simulink library "Copy_of_PTOSim_Lib"  (R2014b)
settings: Solver=ode45  StartTime=0.0  StopTime=10.0  RelTol=1e-3
undefined symbols (not defined in the file or in its folder): pAeq, pAupper_limit, pBeq, pBupper_limit, ptosim, tot
undefined symbols (not defined in the file): valve
settings Model: RequirementInfo="{}  %GIDa_42666abb_d6d9_408c_ae24_f6520282b61c"  Creator=sor  LastModifiedBy=rso

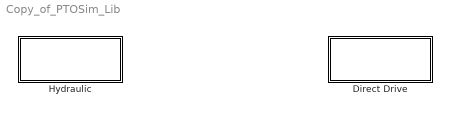
== system Copy_of_PTOSim_Lib ==
  Direct Drive : Subsystem  RequirementInfo="{}  %GIDa_5439fdb4_7c29_433c_8677_23bf92e18f11"
  Hydraulic : Subsystem  RequirementInfo={} %GIDa_f12a42eb_b9cb_4818_b573_b7dee4183a3b

== system Copy_of_PTOSim_Lib/Direct Drive ==
  Electric Machine : Subsystem  RequirementInfo="{}  %GIDa_9a577bd3_d1cd_44c9_a605_4eaf21e33064"  mask{ptosim=ptosim.machine}
      mask prompts: ptosim "Machine Name:"
      mask init:
      | if exist ('ptosim','var')
      |     if ischar(ptosim.Rs)==1 ...
      |        || ischar(ptosim.Bfric)==1 ...
      |        || ischar(ptosim.tau_p)==1 ...
      |        || ischar(ptosim.lambda_fd)==1 ...
      |        || ischar(ptosim.Ls)==1 ...
      |        || ischar(ptosim.theta_d_0)==1 ...
      |        || ischar(ptosim.lambda_sq_0)==1 ...
      |        || ischar(ptosim.lambda_sd_0)==1
      |           error('One of the machine variables is undefined. For example, ptosim.machine.variableName')
      |     end       
      | end
  Load : Subsystem  mask(PTO-Sim Element){ptosim=ptosim.ddload}
      mask prompts: ptosim "Load Name:"
      mask init:
      | if exist ('ptosim','var')
      |     if ischar(ptosim.Rload)==1
      |         error('ptosim.ddload.Rload is undefined')
      |     end
      | end

== system Copy_of_PTOSim_Lib/Hydraulic ==
  Accumulator : Subsystem  mask(PTO-Sim Element){ptosim=ptosim}
      mask prompts: ptosim "Accumulator Name:"
      mask init:
      | if exist('ptosim','var')
      |     if ischar(ptosim.VI0)==1 ...
      |             || ischar(ptosim.pIrated)==1 ...
      |             || ischar(ptosim.pIupper_limit)==1 ...
      |             || ischar(ptosim.pIlower_limit)==1 ...
      |             || ischar(ptosim.pIprecharge)==1 ...
      |             || ischar(ptosim.VImax)==1 ...
      |             || ischar(ptosim.VImin)==1 ...
      |             || ischar(ptosim.VIeq)==1 ...
      |             || ischar(ptosim.pIeq)==1 ...
      |             error('One of the accumulator variable is undefined. For example, ptosim.accum.variableName')
      |     end
      | end
  "Hydraulic Motor " : Subsystem  mask{ptosim=ptosim.motor}
      mask prompts: ptosim "Motor Name:"
      mask init:
      | if exist ('ptosim','var')
      |     if ischar(ptosim.angVelInit)==1 ...
      |        || ischar(ptosim.alpha)==1 ...
      |        || ischar(ptosim.D)==1 ...
      |        || ischar(ptosim.J)==1 ...
      |        || ischar(ptosim.bg)==1 ...
      |        || ischar(ptosim.bf)==1
      |           error('One of the motor variables is undefined. For example, ptosim.motor.variableName')
      |     end       
      | end
  Lookup Table Generator : Subsystem  RequirementInfo="{}  %GIDa_30368e1c_dc2a_4605_bb50_ff3a423f2df5"  mask{ptosim=ptosim.gen}
      mask prompts: ptosim "Generator Name"
      mask init:
      | if exist ('ptosim','var')
      |    if ischar(ptosim.TgenBase)==1 ...
      |       || ischar(ptosim.omegaBase)==1 ...
      |       || ischar(ptosim.driveEff)==1 
      |          error('One of the generator variables is undefined. For example, ptosim.gen.variableName')
      |    end
      | end
  Piston : Subsystem  Variant=on  mask(PTO-Element){piston=ptosim.piston}
      mask prompts: piston "Piston Name:"
  Valve : Subsystem  Variant=on  mask{valve=valve}
      mask prompts: valve "Valve Name"

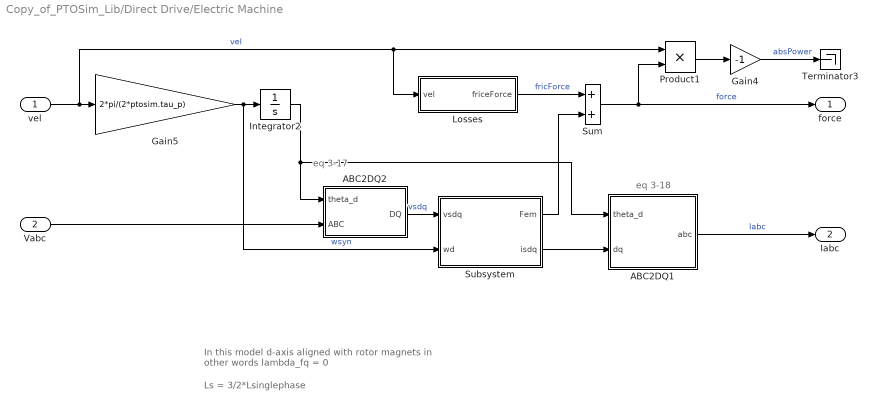
== system Copy_of_PTOSim_Lib/Direct Drive/Electric Machine ==
  note: In this model d-axis aligned with rotor magnets
      | in other words lambda_fq = 0
  note: Ls = 3/2*Lsinglephase
  note: eq 3-17
  note: eq 3-18
  vel : Inport
  Vabc : Inport  Port=2
  ABC2DQ1 : Subsystem
  ABC2DQ2 : Subsystem
  Gain4 : Gain  Gain=-1
  Gain5 : Gain  Gain=2*pi/(2*ptosim.tau_p)
  Integrator2 : Integrator  InitialCondition=ptosim.theta_d_0
  Losses : Subsystem
  Product1 : Product
  Subsystem : Subsystem
  Sum : Sum
  Terminator3 : Terminator
  force : Outport
  Iabc : Outport  Port=2
  wires:
  ABC2DQ2/1(DQ) -> Subsystem/1(vsdq)  "vsdq"
  ABC2DQ1/1(abc) -> Iabc/1  "Iabc"
  vel/1 -> Gain5/1, Losses/1(vel), Product1/1  "vel"
  Gain5/1 -> Subsystem/2(wd), Integrator2/1  "wsyn"
  Integrator2/1 -> ABC2DQ2/1(theta_d), ABC2DQ1/1(theta_d)
  Product1/1 -> Gain4/1
  Gain4/1 -> Terminator3/1  "absPower"
  Subsystem/1(Fem) -> Sum/2
  Vabc/1 -> ABC2DQ2/2(ABC)
  Subsystem/2(isdq) -> ABC2DQ1/2(dq)
  Losses/1(friceForce) -> Sum/1  "fricForce"
  Sum/1 -> Product1/2, force/1  "force"

== system Copy_of_PTOSim_Lib/Direct Drive/Load ==
  Iabc : Inport
  Gain : Gain  Gain=-1
  Gain1 : Gain  Gain=ptosim.Rload
  Product : Product
  Sum of Elements : Sum  Inputs=+
  Vabc : Outport
  elecPower : Outport  Port=2
  wires:
  Gain/1 -> elecPower/1  "elecPower"
  Gain1/1 -> Product/1, Vabc/1  "Vabc"
  Product/1 -> Sum of Elements/1
  Iabc/1 -> Gain1/1, Product/2
  Sum of Elements/1 -> Gain/1

== system Copy_of_PTOSim_Lib/Hydraulic/Accumulator ==
  volFlowM : Inport
  volFlowAccum : Inport  Port=2
  Constant : Constant
  Constant3 : Constant  Value=ptosim.pIprecharge
  Constant4 : Constant  Value=ptosim.VI0
  Divide : Product  Inputs=*/
  Divide1 : Product  Inputs=*/
  Exponent : Constant  Value=1.4
  Integrator4 : Integrator  InitialCondition=ptosim.VIeq
  Math Function : Math  Operator=pow  SaturateOnIntegerOverflow=on
  Sum : Sum  Inputs=-+
  Sum2 : Sum
  pressure : Outport
  wires:
  Sum2/1 -> Integrator4/1
  Integrator4/1 -> Divide/1
  Constant4/1 -> Divide/2
  Constant/1 -> Sum/2
  Divide/1 -> Sum/1
  Exponent/1 -> Math Function/2
  Sum/1 -> Math Function/1
  Math Function/1 -> Divide1/2
  Constant3/1 -> Divide1/1  "pI0"
  Divide1/1 -> pressure/1
  volFlowAccum/1 -> Sum2/2
  volFlowM/1 -> Sum2/1

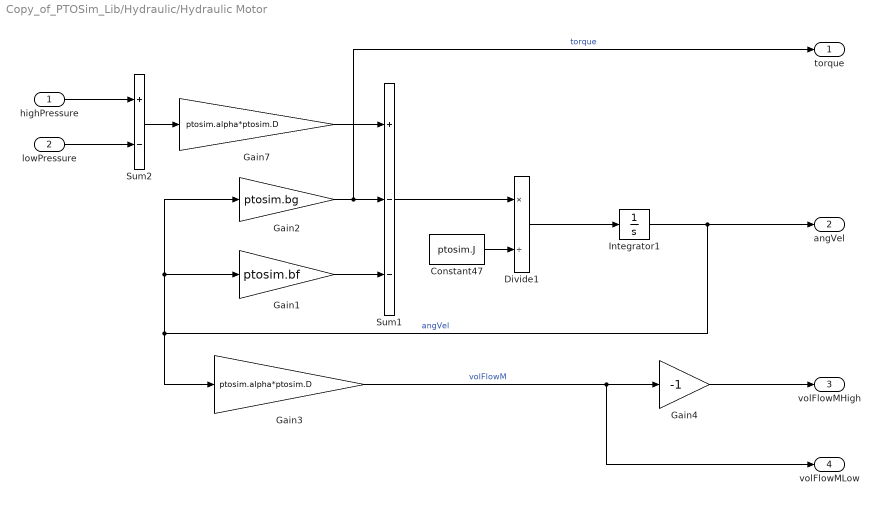
== system Copy_of_PTOSim_Lib/Hydraulic/Hydraulic Motor  ==
  highPressure : Inport
  lowPressure : Inport  Port=2
  Constant47 : Constant  Value=ptosim.J
  Divide1 : Product  Inputs=*/
  Gain1 : Gain  Gain=ptosim.bf
  Gain2 : Gain  Gain=ptosim.bg
  Gain3 : Gain  Gain=ptosim.alpha*ptosim.D
  Gain4 : Gain  Gain=-1
  Gain7 : Gain  Gain=ptosim.alpha*ptosim.D
  Integrator1 : Integrator  InitialCondition=ptosim.angVelInit
  Sum1 : Sum  Inputs=+--
  Sum2 : Sum  Inputs=+-
  torque : Outport
  angVel : Outport  Port=2
  volFlowMHigh : Outport  Port=3
  volFlowMLow : Outport  Port=4
  wires:
  Gain7/1 -> Sum1/1
  Gain2/1 -> torque/1, Sum1/2  "torque"
  Gain1/1 -> Sum1/3
  Sum1/1 -> Divide1/1
  Constant47/1 -> Divide1/2
  Divide1/1 -> Integrator1/1
  Integrator1/1 -> angVel/1, Gain3/1, Gain2/1, Gain1/1  "angVel"
  Gain3/1 -> volFlowMLow/1, Gain4/1  "volFlowM"
  highPressure/1 -> Sum2/1
  lowPressure/1 -> Sum2/2
  Sum2/1 -> Gain7/1
  Gain4/1 -> volFlowMHigh/1

== system Copy_of_PTOSim_Lib/Hydraulic/Lookup Table Generator ==
  torque : Inport
  angVel : Inport  Port=2
  Base Motor Torque : Gain  Gain=-1/ptosim.TgenBase
  Base Motor Torque1 : Gain  Gain=1/ptosim.omegaBase
  Base Motor Torque2 : Gain  Gain=ptosim.driveEff
  Base Motor Torque3 : Gain  Gain=1/100
  PM p.u. Efficiency Lookup Table : Lookup_n-D  BreakpointsForDimension1=tot.Tpu(:,1)  BreakpointsForDimension2=tot.omegapu(1,:)  Table=tot.eff  InterpMethod=Flat  InputSameDT=on
  Product : Product  RndMeth=Zero
  Product1 : Product  RndMeth=Zero
  elecPower : Outport
  wires:
  Base Motor Torque2/1 -> elecPower/1  "elecPower"
  Product1/1 -> Base Motor Torque2/1
  Product/1 -> Product1/1  "genPower"
  Base Motor Torque3/1 -> Product1/2  "genEff"
  PM p.u. Efficiency Lookup Table/1 -> Base Motor Torque3/1
  angVel/1 -> Product/2, Base Motor Torque1/1
  Base Motor Torque1/1 -> PM p.u. Efficiency Lookup Table/2  "omegaPU"
  torque/1 -> Product/1, Base Motor Torque/1
  Base Motor Torque/1 -> PM p.u. Efficiency Lookup Table/1  "torquePU"

== system Copy_of_PTOSim_Lib/Hydraulic/Piston ==
  note: 1) Add Subsystem or Model blocks as valid variant choices.
      | 2) You cannot connect blocks at this level. At simulation, connectivity is automatically
      | determined, based on the active variant and port name matching.
  response : Inport
  volFlowC : Inport  Port=2
  pressureNC : Inport  Port=3
  PistonC : Subsystem  VariantControl=compressFluid  mask{ptosim=ptosim.piston}
      mask prompts: ptosim "Piston Name:"
      mask init:
      | if exist ('ptosim','var')
      |     if ischar(ptosim.Ap)==1 ...
      |       || ischar(ptosim.Vo)==1 ...
      |       || ischar(ptosim.Beta_e)==1 ...
      |       || ischar(ptosim.pAi)==1 ...
      |       || ischar(ptosim.pBi)==1 
      |          error('One of the piston variable is undefined. For example, ptosim.piston.variableName')    
      |     end
      | end
  PistonNC : Subsystem  VariantControl=noncompressFluid  mask(PTO-Sim Element){ptosim=ptosim.piston}
      mask prompts: ptosim "Piston Name:"
      mask init:
      | if exist ('ptosim','var')
      |     if ischar(ptosim.topA)==1 ...
      |       || ischar(ptosim.botA)==1
      |          error('One of the piston variables is undefined. For example, ptosim.piston.variableName')
      |     end
      | end
  force : Outport
  pressureC : Outport  Port=2
  volFlowNC : Outport  Port=3

== system Copy_of_PTOSim_Lib/Hydraulic/Valve ==
  note: 1) Add Subsystem or Model blocks as valid variant choices.
      | 2) You cannot connect blocks at this level. At simulation, connectivity is automatically
      | determined, based on the active variant and port name matching.
  pressureC : Inport
  volFlowNC : Inport  Port=2
  ValveC : Subsystem  VariantControl=compressFluid  mask{ptosim=ptosim.valve}
      mask prompts: ptosim "Valve Name:"
      mask init:
      | if exist ('ptosim','var')
      |     if ischar(ptosim.Cd)==1 ...
      |        || ischar(ptosim.Amax)==1 ...
      |        || ischar(ptosim.Amin)==1 ...
      |        || ischar(ptosim.pMax)==1 ...
      |        || ischar(ptosim.pMin)==1 ...
      |        || ischar(ptosim.rho)==1 ...
      |        || ischar(ptosim.k1)==1 ...
      |        || ischar(ptosim.k2)==1 
      |           error('One of valve variables is undefined. For exmaple, ptosim.valve.variableName')
      |     end
      | end
  ValveNC : Subsystem  VariantControl=noncompressFluid  mask(PTO-Sim Element){ptosim=0}
      mask prompts: ptosim "Valve Name:"
  volFlow : Outport

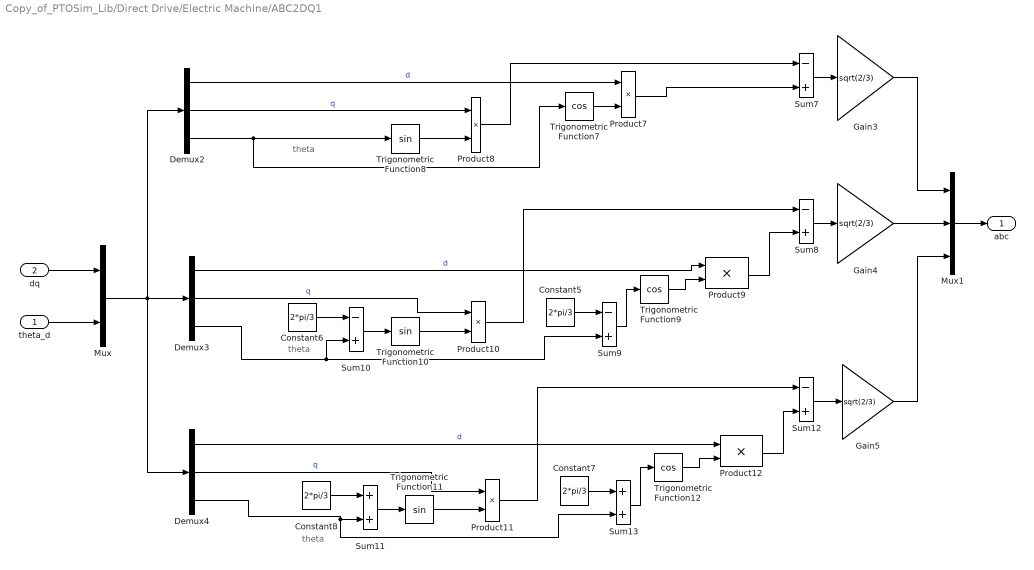
== system Copy_of_PTOSim_Lib/Direct Drive/Electric Machine/ABC2DQ1 ==
  note: theta
  note: theta
  note: theta
  theta_d : Inport
  dq : Inport  Port=2
  Constant{5..8} (4 alike) : Constant  Value=2*pi/3
  Demux2 : Demux  Outputs=3
  Demux3 : Demux  Outputs=3
  Demux4 : Demux  Outputs=3
  Gain3 : Gain  Gain=sqrt(2/3)  SaturateOnIntegerOverflow=on  OutDataTypeStr=Inherit: Same as input  ParamDataTypeStr=Inherit: Same as input
  Gain4 : Gain  Gain=sqrt(2/3)  SaturateOnIntegerOverflow=on  OutDataTypeStr=Inherit: Same as input  ParamDataTypeStr=Inherit: Same as input
  Gain5 : Gain  Gain=sqrt(2/3)  SaturateOnIntegerOverflow=on  OutDataTypeStr=Inherit: Same as input  ParamDataTypeStr=Inherit: Same as input
  Mux : Mux  Inputs=2
  Mux1 : Mux  Inputs=3
  Product{7..12} (6 alike) : Product  SaturateOnIntegerOverflow=on  InputSameDT=on  OutDataTypeStr=Inherit: Same as first input
  Sum{7..10,12} (5 alike) : Sum  Inputs=-+  SaturateOnIntegerOverflow=on  InputSameDT=on  OutDataTypeStr=Inherit: Same as first input
  Sum11 : Sum  SaturateOnIntegerOverflow=on  InputSameDT=on  OutDataTypeStr=Inherit: Same as first input
  Sum13 : Sum  SaturateOnIntegerOverflow=on  InputSameDT=on  OutDataTypeStr=Inherit: Same as first input
  Trigonometric Function10 : Trigonometry
  Trigonometric Function11 : Trigonometry
  Trigonometric Function12 : Trigonometry  Operator=cos
  Trigonometric Function7 : Trigonometry  Operator=cos
  Trigonometric Function8 : Trigonometry
  Trigonometric Function9 : Trigonometry  Operator=cos
  abc : Outport
  wires:
  Mux1/1 -> abc/1
  dq/1 -> Mux/1
  theta_d/1 -> Mux/2
  Mux/1 -> Demux4/1, Demux2/1, Demux3/1
  Trigonometric Function7/1 -> Product7/2
  Demux2/1 -> Product7/1  "d"
  Product7/1 -> Sum7/2
  Product8/1 -> Sum7/1
  Demux2/3 -> Trigonometric Function8/1, Trigonometric Function7/1
  Demux2/2 -> Product8/1  "q"
  Trigonometric Function9/1 -> Product9/2
  Demux3/1 -> Product9/1  "d"
  Product9/1 -> Sum8/2
  Product10/1 -> Sum8/1
  Demux3/3 -> Sum10/2, Sum9/2
  Trigonometric Function10/1 -> Product10/2
  Demux3/2 -> Product10/1  "q"
  Sum9/1 -> Trigonometric Function9/1
  Constant5/1 -> Sum9/1
  Sum10/1 -> Trigonometric Function10/1
  Constant6/1 -> Sum10/1
  Trigonometric Function12/1 -> Product12/2
  Demux4/1 -> Product12/1  "d"
  Product12/1 -> Sum12/2
  Product11/1 -> Sum12/1
  Demux4/3 -> Sum13/2, Sum11/2
  Trigonometric Function11/1 -> Product11/2
  Demux4/2 -> Product11/1  "q"
  Sum13/1 -> Trigonometric Function12/1
  Constant7/1 -> Sum13/1
  Sum11/1 -> Trigonometric Function11/1
  Constant8/1 -> Sum11/1
  Sum7/1 -> Gain3/1
  Sum8/1 -> Gain4/1
  Sum12/1 -> Gain5/1
  Gain3/1 -> Mux1/1
  Gain4/1 -> Mux1/2
  Gain5/1 -> Mux1/3
  Trigonometric Function8/1 -> Product8/2

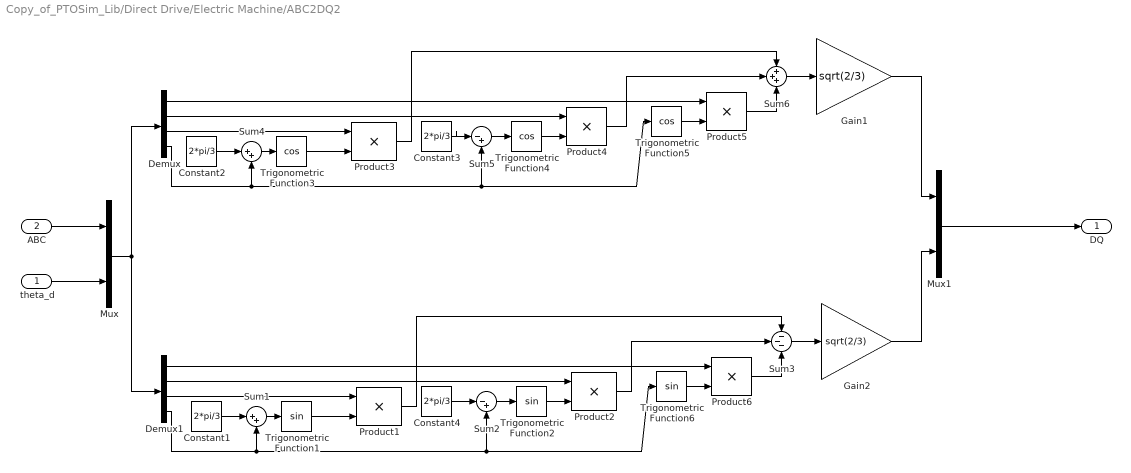
== system Copy_of_PTOSim_Lib/Direct Drive/Electric Machine/ABC2DQ2 ==
  theta_d : Inport
  ABC : Inport  Port=2
  Constant{1..4} (4 alike) : Constant  Value=2*pi/3
  Demux : Demux
  Demux1 : Demux
  Gain1 : Gain  Gain=sqrt(2/3)  SaturateOnIntegerOverflow=on  OutDataTypeStr=Inherit: Same as input  ParamDataTypeStr=Inherit: Same as input
  Gain2 : Gain  Gain=sqrt(2/3)  SaturateOnIntegerOverflow=on  OutDataTypeStr=Inherit: Same as input  ParamDataTypeStr=Inherit: Same as input
  Mux : Mux  Inputs=2
  Mux1 : Mux  Inputs=2
  Product{1..6} (6 alike) : Product  SaturateOnIntegerOverflow=on  InputSameDT=on  OutDataTypeStr=Inherit: Same as first input
  Sum1 : Sum  Inputs=|++  SaturateOnIntegerOverflow=on  InputSameDT=on  OutDataTypeStr=Inherit: Same as first input
  Sum2 : Sum  Inputs=|-+  SaturateOnIntegerOverflow=on  InputSameDT=on  OutDataTypeStr=Inherit: Same as first input
  Sum3 : Sum  Inputs=---  SaturateOnIntegerOverflow=on  InputSameDT=on  OutDataTypeStr=Inherit: Same as first input
  Sum4 : Sum  Inputs=|++  SaturateOnIntegerOverflow=on  InputSameDT=on  OutDataTypeStr=Inherit: Same as first input
  Sum5 : Sum  Inputs=|-+  SaturateOnIntegerOverflow=on  InputSameDT=on  OutDataTypeStr=Inherit: Same as first input
  Sum6 : Sum  Inputs=+++  SaturateOnIntegerOverflow=on  InputSameDT=on  OutDataTypeStr=Inherit: Same as first input
  Trigonometric Function1 : Trigonometry
  Trigonometric Function2 : Trigonometry
  Trigonometric Function3 : Trigonometry  Operator=cos
  Trigonometric Function4 : Trigonometry  Operator=cos
  Trigonometric Function5 : Trigonometry  Operator=cos
  Trigonometric Function6 : Trigonometry
  DQ : Outport
  wires:
  Mux1/1 -> DQ/1
  Product5/1 -> Sum6/3
  Constant2/1 -> Sum4/1
  Sum5/1 -> Trigonometric Function4/1
  Trigonometric Function4/1 -> Product4/2
  Trigonometric Function5/1 -> Product5/2
  Constant3/1 -> Sum5/1
  Sum6/1 -> Gain1/1
  Product3/1 -> Sum6/1
  Product4/1 -> Sum6/2
  Trigonometric Function3/1 -> Product3/2
  Gain1/1 -> Mux1/1
  ABC/1 -> Mux/1
  theta_d/1 -> Mux/2
  Demux/1 -> Product5/1
  Demux/2 -> Product4/1
  Demux/3 -> Product3/1
  Demux/4 -> Sum5/2, Trigonometric Function5/1, Sum4/2
  Mux/1 -> Demux/1, Demux1/1
  Sum4/1 -> Trigonometric Function3/1
  Product6/1 -> Sum3/3
  Constant1/1 -> Sum1/1
  Sum2/1 -> Trigonometric Function2/1
  Trigonometric Function2/1 -> Product2/2
  Trigonometric Function6/1 -> Product6/2
  Constant4/1 -> Sum2/1
  Sum3/1 -> Gain2/1
  Product1/1 -> Sum3/1
  Product2/1 -> Sum3/2
  Trigonometric Function1/1 -> Product1/2
  Gain2/1 -> Mux1/2
  Demux1/1 -> Product6/1
  Demux1/2 -> Product2/1
  Demux1/3 -> Product1/1
  Demux1/4 -> Sum1/2, Trigonometric Function6/1, Sum2/2
  Sum1/1 -> Trigonometric Function1/1

== system Copy_of_PTOSim_Lib/Direct Drive/Electric Machine/Losses ==
  vel : Inport
  Gain : Gain  Gain=ptosim.Bfric
  friceForce : Outport
  wires:
  vel/1 -> Gain/1
  Gain/1 -> friceForce/1

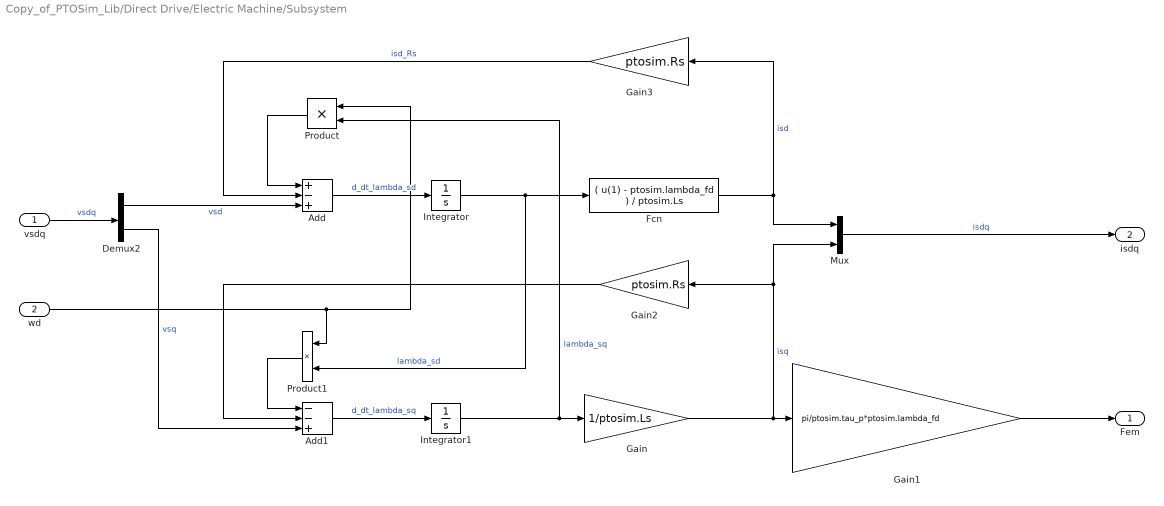
== system Copy_of_PTOSim_Lib/Direct Drive/Electric Machine/Subsystem ==
  vsdq : Inport
  wd : Inport  Port=2
  Add : Sum  Inputs=+-+
  Add1 : Sum  Inputs=--+
  Demux2 : Demux  Outputs=2
  Fcn : Fcn  Expr=( u(1) - ptosim.lambda_fd ) / ptosim.Ls
  Gain : Gain  Gain=1/ptosim.Ls
  Gain1 : Gain  Gain=pi/ptosim.tau_p*ptosim.lambda_fd
  Gain2 : Gain  Gain=ptosim.Rs
  Gain3 : Gain  Gain=ptosim.Rs
  Integrator : Integrator  InitialCondition=ptosim.lambda_sd_0
  Integrator1 : Integrator  InitialCondition=ptosim.lambda_sq_0
  Mux : Mux  Inputs=2
  Product : Product  RndMeth=Zero
  Product1 : Product  RndMeth=Zero
  Fem : Outport
  isdq : Outport  Port=2
  wires:
  Add/1 -> Integrator/1  "d_dt_lambda_sd"
  Integrator/1 -> Product1/2, Fcn/1  "lambda_sd"
  Fcn/1 -> Gain3/1, Mux/1  "isd"
  Product/1 -> Add/1
  Add1/1 -> Integrator1/1  "d_dt_lambda_sq"
  Integrator1/1 -> Gain/1, Product/2  "lambda_sq"
  wd/1 -> Product1/1, Product/1
  Gain/1 -> Gain2/1, Mux/2, Gain1/1  "isq"
  Product1/1 -> Add1/1
  Demux2/1 -> Add/3  "vsd"
  Demux2/2 -> Add1/3  "vsq"
  vsdq/1 -> Demux2/1  "vsdq"
  Gain3/1 -> Add/2  "isd_Rs"
  Gain2/1 -> Add1/2
  Mux/1 -> isdq/1  "isdq"
  Gain1/1 -> Fem/1

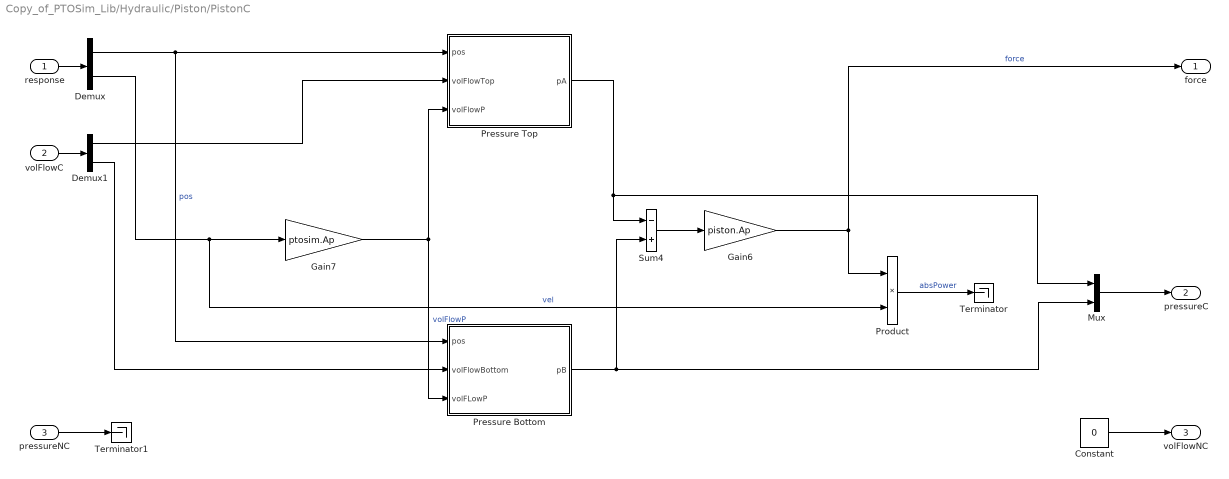
== system Copy_of_PTOSim_Lib/Hydraulic/Piston/PistonC ==
  response : Inport
  volFlowC : Inport  Port=2
  pressureNC : Inport  Port=3
  Constant : Constant  Value=0
  Demux : Demux  Outputs=2
  Demux1 : Demux  Outputs=2
  Gain6 : Gain  Gain=piston.Ap
  Gain7 : Gain  Gain=ptosim.Ap
  Mux : Mux  Inputs=2
  Pressure Bottom : Subsystem
  Pressure Top : Subsystem
  Product : Product
  Sum4 : Sum  Inputs=-+
  Terminator : Terminator
  Terminator1 : Terminator
  force : Outport
  pressureC : Outport  Port=2
  volFlowNC : Outport  Port=3
  wires:
  Pressure Top/1(pA) -> Mux/1, Sum4/1
  Pressure Bottom/1(pB) -> Mux/2, Sum4/2
  Gain7/1 -> Pressure Bottom/3(volFLowP), Pressure Top/3(volFlowP)  "volFlowP"
  Product/1 -> Terminator/1  "absPower"
  Demux/1 -> Pressure Bottom/1(pos), Pressure Top/1(pos)  "pos"
  Demux/2 -> Product/2, Gain7/1  "vel"
  Sum4/1 -> Gain6/1
  Gain6/1 -> force/1, Product/1  "force"
  Demux1/1 -> Pressure Top/2(volFlowTop)
  Demux1/2 -> Pressure Bottom/2(volFlowBottom)
  response/1 -> Demux/1
  volFlowC/1 -> Demux1/1
  Mux/1 -> pressureC/1
  Constant/1 -> volFlowNC/1
  pressureNC/1 -> Terminator1/1

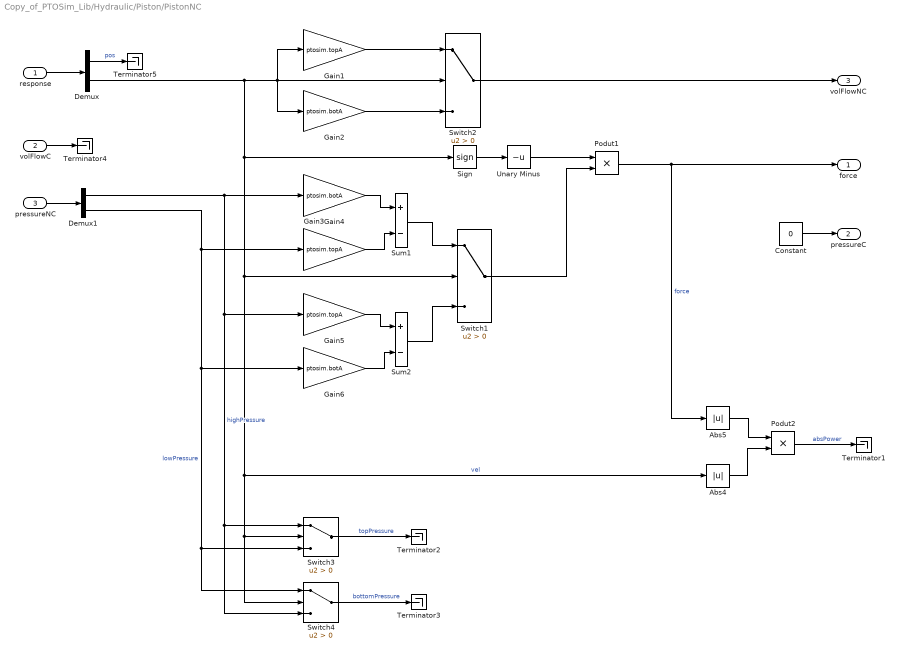
== system Copy_of_PTOSim_Lib/Hydraulic/Piston/PistonNC ==
  response : Inport
  volFlowC : Inport  Port=2
  pressureNC : Inport  Port=3
  Abs4 : Abs
  Abs5 : Abs
  Constant : Constant  Value=0
  Demux : Demux  Outputs=2
  Demux1 : Demux  Outputs=2
  Gain1 : Gain  Gain=ptosim.topA
  Gain2 : Gain  Gain=ptosim.botA
  Gain3 : Gain  Gain=ptosim.topA
  Gain4 : Gain  Gain=ptosim.botA
  Gain5 : Gain  Gain=ptosim.topA
  Gain6 : Gain  Gain=ptosim.botA
  Podut1 : Product  RndMeth=Zero
  Podut2 : Product  RndMeth=Zero
  Sign : Signum
  Sum1 : Sum  Inputs=+-
  Sum2 : Sum  Inputs=+-
  Switch{1..4} (4 alike) : Switch  Criteria=u2 > Threshold
  Terminator{1..5} (5 alike) : Terminator
  Unary Minus : UnaryMinus
  force : Outport
  pressureC : Outport  Port=2
  volFlowNC : Outport  Port=3
  wires:
  Demux/2 -> Switch1/2, Switch4/2, Switch3/2, Abs4/1, Sign/1, Gain2/1, Switch2/2, Gain1/1  "vel"
  Podut2/1 -> Terminator1/1  "absPower"
  Abs5/1 -> Podut2/1
  Abs4/1 -> Podut2/2
  Gain1/1 -> Switch2/1
  Gain2/1 -> Switch2/3
  Switch2/1 -> volFlowNC/1
  Sum1/1 -> Switch1/1
  Podut1/1 -> Abs5/1, force/1  "force"
  Gain4/1 -> Sum1/1
  Gain3/1 -> Sum1/2
  Demux1/1 -> Gain5/1, Switch3/1, Switch4/3, Gain4/1  "highPressure"
  Demux1/2 -> Switch4/1, Switch3/3, Gain6/1, Gain3/1  "lowPressure"
  Gain5/1 -> Sum2/1
  Gain6/1 -> Sum2/2
  Sum2/1 -> Switch1/3
  Sign/1 -> Unary Minus/1
  Unary Minus/1 -> Podut1/1
  Switch1/1 -> Podut1/2
  Switch3/1 -> Terminator2/1  "topPressure"
  Switch4/1 -> Terminator3/1  "bottomPressure"
  response/1 -> Demux/1
  volFlowC/1 -> Terminator4/1
  pressureNC/1 -> Demux1/1
  Demux/1 -> Terminator5/1  "pos"
  Constant/1 -> pressureC/1

== system Copy_of_PTOSim_Lib/Hydraulic/Valve/ValveC ==
  pressureC : Inport
  volFlowNC : Inport  Port=2
  Demux : Demux
  Mux : Mux
  Subsystem : Subsystem  RequirementInfo="{}  %GIDa_43e7490a_26e5_4c96_a755_05599e7ab58d"
  Subsystem1 : Subsystem
  Subsystem2 : Subsystem
  Subsystem3 : Subsystem  RequirementInfo="{}  %GIDa_1d14c02d_1c58_4958_a821_20fe782ea22d"
  Sum1 : Sum  Inputs=-+
  Sum2 : Sum
  Sum3 : Sum  Inputs=--
  Sum4 : Sum  Inputs=-+
  Terminator : Terminator
  volFlow : Outport
  wires:
  Demux/1 -> Subsystem/1(topPressure), Subsystem3/2(topPressure)  "topPressure"
  Demux/2 -> Subsystem1/1(bottomPressure), Subsystem2/2(bottomPressure)  "bottomPressure"
  Demux/3 -> Subsystem1/2(highPressure), Subsystem/2(highPressure)  "highPressure"
  Demux/4 -> Subsystem3/1(lowPressure), Subsystem2/1(lowPressure)  "lowPressure"
  Subsystem3/1(volFlow4) -> Sum4/2, Sum3/2  "volFlow4"
  Subsystem2/1(volFlow3) -> Sum3/1, Sum1/2  "volFlow3"
  Subsystem1/1(volFlow2) -> Sum2/2, Sum1/1  "volFlow2"
  Subsystem/1(volFlow1) -> Sum2/1, Sum4/1  "volFlow1"
  Sum4/1 -> Mux/1  "volFlowTop"
  Sum1/1 -> Mux/2  "volFlowBottom"
  Sum2/1 -> Mux/3  "volFlowHigh"
  Sum3/1 -> Mux/4  "volFlowLow"
  pressureC/1 -> Demux/1
  volFlowNC/1 -> Terminator/1
  Mux/1 -> volFlow/1

== system Copy_of_PTOSim_Lib/Hydraulic/Valve/ValveNC ==
  pressureC : Inport
  volFlowNC : Inport  Port=2
  Abs1 : Abs
  Mux : Mux  Inputs=2
  Terminator : Terminator
  electric generator control1 : Gain  Gain=-1
  volFlow : Outport
  wires:
  Abs1/1 -> electric generator control1/1, Mux/1  "volFlow"
  electric generator control1/1 -> Mux/2
  volFlowNC/1 -> Abs1/1
  pressureC/1 -> Terminator/1
  Mux/1 -> volFlow/1

== system Copy_of_PTOSim_Lib/Hydraulic/Piston/PistonC/Pressure Bottom ==
  pos : Inport
  volFlowBottom : Inport  Port=2
  volFLowP : Inport  Port=3
  Constant1 : Constant  Value=ptosim.Vo
  Divide1 : Product  Inputs=*/
  Gain4 : Gain  Gain=ptosim.Beta_e
  Gain5 : Gain  Gain=ptosim.Ap
  Integrator3 : Integrator  InitialCondition=ptosim.pBi  UpperSaturationLimit=pBupper_limit  LowerSaturationLimit=pBeq
  Sum2 : Sum  Inputs=+-
  Sum3 : Sum
  pB : Outport
  wires:
  volFLowP/1 -> Sum2/2
  Integrator3/1 -> pB/1
  volFlowBottom/1 -> Sum2/1
  Divide1/1 -> Integrator3/1  "pBdot"
  Sum3/1 -> Divide1/2
  Gain4/1 -> Divide1/1
  Constant1/1 -> Sum3/2
  Gain5/1 -> Sum3/1
  pos/1 -> Gain5/1
  Sum2/1 -> Gain4/1

== system Copy_of_PTOSim_Lib/Hydraulic/Piston/PistonC/Pressure Top ==
  pos : Inport
  volFlowTop : Inport  Port=2
  volFlowP : Inport  Port=3
  Constant : Constant  Value=ptosim.Vo
  Divide : Product  Inputs=*/
  Gain1 : Gain  Gain=ptosim.Beta_e
  Gain2 : Gain  Gain=ptosim.Ap
  Integrator2 : Integrator  InitialCondition=ptosim.pAi  UpperSaturationLimit=pAupper_limit  LowerSaturationLimit=pAeq
  Sum : Sum
  Sum1 : Sum  Inputs=-+
  pA : Outport
  wires:
  volFlowP/1 -> Sum/2
  Integrator2/1 -> pA/1
  Divide/1 -> Integrator2/1  "pAdot"
  volFlowTop/1 -> Sum/1
  Sum1/1 -> Divide/2
  Gain1/1 -> Divide/1
  Constant/1 -> Sum1/2
  Gain2/1 -> Sum1/1
  pos/1 -> Gain2/1
  Sum/1 -> Gain1/1

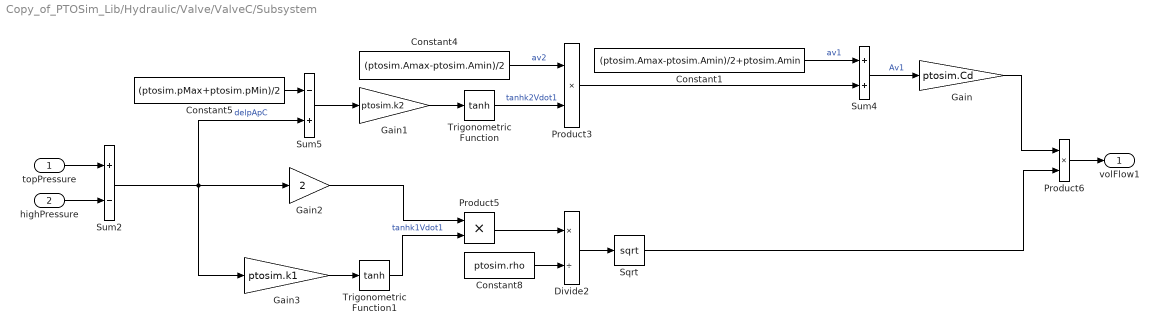
== system Copy_of_PTOSim_Lib/Hydraulic/Valve/ValveC/Subsystem ==
  topPressure : Inport
  highPressure : Inport  Port=2
  Constant1 : Constant  Value=(ptosim.Amax-ptosim.Amin)/2+ptosim.Amin
  Constant4 : Constant  Value=(ptosim.Amax-ptosim.Amin)/2
  Constant5 : Constant  Value=(ptosim.pMax+ptosim.pMin)/2
  Constant8 : Constant  Value=ptosim.rho
  Divide2 : Product  Inputs=*/
  Gain : Gain  Gain=ptosim.Cd
  Gain1 : Gain  Gain=ptosim.k2
  Gain2 : Gain  Gain=2
  Gain3 : Gain  Gain=ptosim.k1
  Product3 : Product
  Product5 : Product
  Product6 : Product
  Sqrt : Sqrt  SaturateOnIntegerOverflow=on
  Sum2 : Sum  Inputs=+-
  Sum4 : Sum
  Sum5 : Sum  Inputs=-+
  Trigonometric Function : Trigonometry  Operator=tanh
  Trigonometric Function1 : Trigonometry  Operator=tanh
  volFlow1 : Outport
  wires:
  Gain1/1 -> Trigonometric Function/1
  Trigonometric Function/1 -> Product3/2  "tanhk2Vdot1"
  Product3/1 -> Sum4/2
  Sum5/1 -> Gain1/1
  Sum4/1 -> Gain/1  "Av1"
  Gain3/1 -> Trigonometric Function1/1
  Gain2/1 -> Product5/1
  Trigonometric Function1/1 -> Product5/2  "tanhk1Vdot1"
  Sqrt/1 -> Product6/2
  Gain/1 -> Product6/1
  Constant8/1 -> Divide2/2
  Product5/1 -> Divide2/1
  Divide2/1 -> Sqrt/1
  topPressure/1 -> Sum2/1
  highPressure/1 -> Sum2/2
  Product6/1 -> volFlow1/1
  Constant4/1 -> Product3/1  "av2"
  Constant5/1 -> Sum5/1
  Constant1/1 -> Sum4/1  "av1"
  Sum2/1 -> Gain3/1, Sum5/2, Gain2/1  "delpApC"

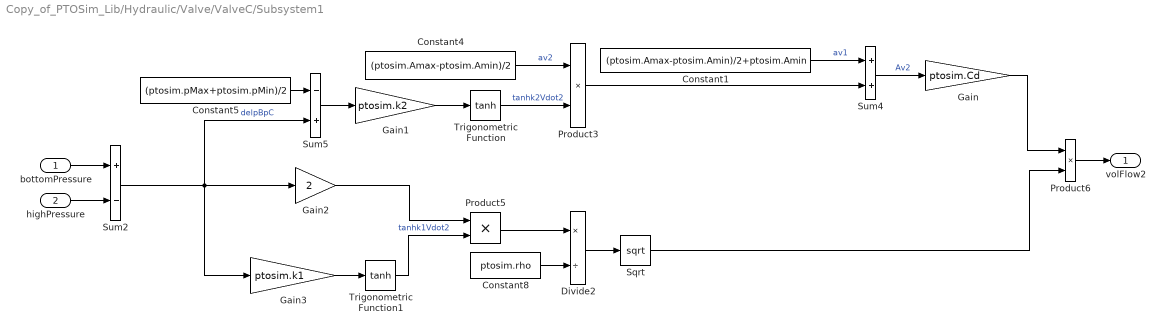
== system Copy_of_PTOSim_Lib/Hydraulic/Valve/ValveC/Subsystem1 ==
  bottomPressure : Inport
  highPressure : Inport  Port=2
  Constant1 : Constant  Value=(ptosim.Amax-ptosim.Amin)/2+ptosim.Amin
  Constant4 : Constant  Value=(ptosim.Amax-ptosim.Amin)/2
  Constant5 : Constant  Value=(ptosim.pMax+ptosim.pMin)/2
  Constant8 : Constant  Value=ptosim.rho
  Divide2 : Product  Inputs=*/
  Gain : Gain  Gain=ptosim.Cd
  Gain1 : Gain  Gain=ptosim.k2
  Gain2 : Gain  Gain=2
  Gain3 : Gain  Gain=ptosim.k1
  Product3 : Product
  Product5 : Product
  Product6 : Product
  Sqrt : Sqrt  SaturateOnIntegerOverflow=on
  Sum2 : Sum  Inputs=+-
  Sum4 : Sum
  Sum5 : Sum  Inputs=-+
  Trigonometric Function : Trigonometry  Operator=tanh
  Trigonometric Function1 : Trigonometry  Operator=tanh
  volFlow2 : Outport
  wires:
  Gain1/1 -> Trigonometric Function/1
  Trigonometric Function/1 -> Product3/2  "tanhk2Vdot2"
  Product3/1 -> Sum4/2
  Sum5/1 -> Gain1/1
  Sum4/1 -> Gain/1  "Av2"
  Gain3/1 -> Trigonometric Function1/1
  Gain2/1 -> Product5/1
  Trigonometric Function1/1 -> Product5/2  "tanhk1Vdot2"
  Sqrt/1 -> Product6/2
  Gain/1 -> Product6/1
  Constant8/1 -> Divide2/2
  Product5/1 -> Divide2/1
  Divide2/1 -> Sqrt/1
  bottomPressure/1 -> Sum2/1
  highPressure/1 -> Sum2/2
  Product6/1 -> volFlow2/1
  Constant4/1 -> Product3/1  "av2"
  Constant5/1 -> Sum5/1
  Constant1/1 -> Sum4/1  "av1"
  Sum2/1 -> Gain3/1, Sum5/2, Gain2/1  "delpBpC"

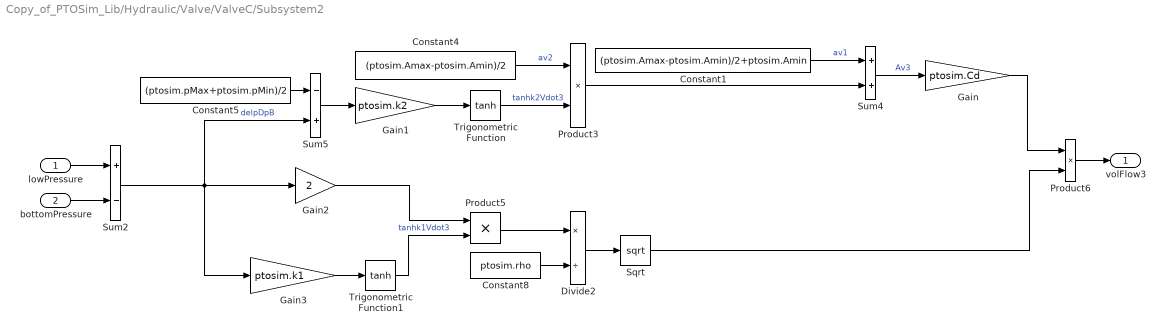
== system Copy_of_PTOSim_Lib/Hydraulic/Valve/ValveC/Subsystem2 ==
  lowPressure : Inport
  bottomPressure : Inport  Port=2
  Constant1 : Constant  Value=(ptosim.Amax-ptosim.Amin)/2+ptosim.Amin
  Constant4 : Constant  Value=(ptosim.Amax-ptosim.Amin)/2
  Constant5 : Constant  Value=(ptosim.pMax+ptosim.pMin)/2
  Constant8 : Constant  Value=ptosim.rho
  Divide2 : Product  Inputs=*/
  Gain : Gain  Gain=ptosim.Cd
  Gain1 : Gain  Gain=ptosim.k2
  Gain2 : Gain  Gain=2
  Gain3 : Gain  Gain=ptosim.k1
  Product3 : Product
  Product5 : Product
  Product6 : Product
  Sqrt : Sqrt  SaturateOnIntegerOverflow=on
  Sum2 : Sum  Inputs=+-
  Sum4 : Sum
  Sum5 : Sum  Inputs=-+
  Trigonometric Function : Trigonometry  Operator=tanh
  Trigonometric Function1 : Trigonometry  Operator=tanh
  volFlow3 : Outport
  wires:
  Gain1/1 -> Trigonometric Function/1
  Trigonometric Function/1 -> Product3/2  "tanhk2Vdot3"
  Product3/1 -> Sum4/2
  Sum5/1 -> Gain1/1
  Sum4/1 -> Gain/1  "Av3"
  Gain3/1 -> Trigonometric Function1/1
  Gain2/1 -> Product5/1
  Trigonometric Function1/1 -> Product5/2  "tanhk1Vdot3"
  Sqrt/1 -> Product6/2
  Gain/1 -> Product6/1
  Constant8/1 -> Divide2/2
  Product5/1 -> Divide2/1
  Divide2/1 -> Sqrt/1
  lowPressure/1 -> Sum2/1
  bottomPressure/1 -> Sum2/2
  Product6/1 -> volFlow3/1
  Constant4/1 -> Product3/1  "av2"
  Constant5/1 -> Sum5/1
  Constant1/1 -> Sum4/1  "av1"
  Sum2/1 -> Gain3/1, Sum5/2, Gain2/1  "delpDpB"

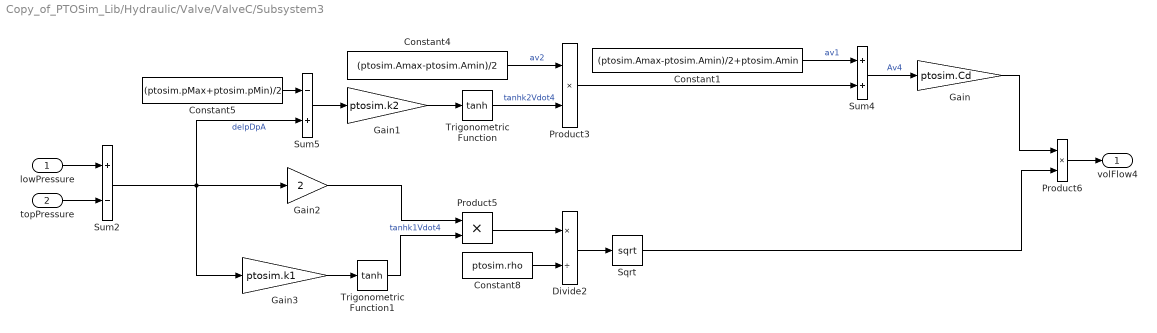
== system Copy_of_PTOSim_Lib/Hydraulic/Valve/ValveC/Subsystem3 ==
  lowPressure : Inport
  topPressure : Inport  Port=2
  Constant1 : Constant  Value=(ptosim.Amax-ptosim.Amin)/2+ptosim.Amin
  Constant4 : Constant  Value=(ptosim.Amax-ptosim.Amin)/2
  Constant5 : Constant  Value=(ptosim.pMax+ptosim.pMin)/2
  Constant8 : Constant  Value=ptosim.rho
  Divide2 : Product  Inputs=*/
  Gain : Gain  Gain=ptosim.Cd
  Gain1 : Gain  Gain=ptosim.k2
  Gain2 : Gain  Gain=2
  Gain3 : Gain  Gain=ptosim.k1
  Product3 : Product
  Product5 : Product
  Product6 : Product
  Sqrt : Sqrt  SaturateOnIntegerOverflow=on
  Sum2 : Sum  Inputs=+-
  Sum4 : Sum
  Sum5 : Sum  Inputs=-+
  Trigonometric Function : Trigonometry  Operator=tanh
  Trigonometric Function1 : Trigonometry  Operator=tanh
  volFlow4 : Outport
  wires:
  Gain1/1 -> Trigonometric Function/1
  Trigonometric Function/1 -> Product3/2  "tanhk2Vdot4"
  Product3/1 -> Sum4/2
  Sum5/1 -> Gain1/1
  Sum4/1 -> Gain/1  "Av4"
  Gain3/1 -> Trigonometric Function1/1
  Gain2/1 -> Product5/1
  Trigonometric Function1/1 -> Product5/2  "tanhk1Vdot4"
  Sqrt/1 -> Product6/2
  Gain/1 -> Product6/1
  Constant8/1 -> Divide2/2
  Product5/1 -> Divide2/1
  Divide2/1 -> Sqrt/1
  lowPressure/1 -> Sum2/1
  topPressure/1 -> Sum2/2
  Product6/1 -> volFlow4/1
  Constant4/1 -> Product3/1  "av2"
  Constant5/1 -> Sum5/1
  Constant1/1 -> Sum4/1  "av1"
  Sum2/1 -> Gain3/1, Sum5/2, Gain2/1  "delpDpA"
